simulink model "SlidesExampleNew_example"  (Simulink 7.4)
settings: Solver=FixedStepDiscrete  StartTime=0.0  StopTime=120  FixedStep=0.5  MaxStep=1  RelTol=1e-3
values from neighbouring files (symbols this model uses):
  y0 = -20    [SlidesExampleMfile.m]    (also in TrajectoryExampleScript.m)
libraries: BLOM_Lib x5
settings Model: Creator=vichik  LastModifiedBy=Kyle
settings OptimizationCC: BlockReduction=off  InitFltsAndDblsToZero=on
settings DebuggingCC: StrictBusMsg=ErrorLevel1

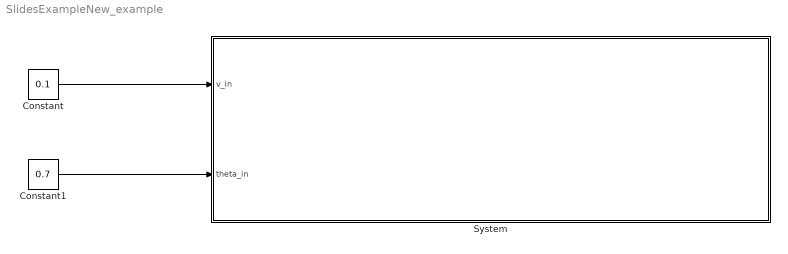
== system SlidesExampleNew_example ==
  Constant : Constant  Value=0.1
  Constant1 : Constant  Value=0.7
  System : Subsystem
  wires:
  Constant/1 -> System/1(v_in)
  Constant1/1 -> System/2(theta_in)

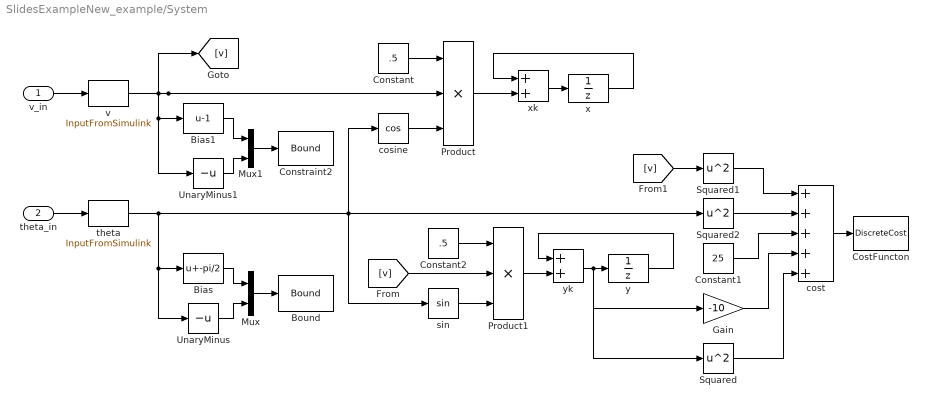
== system SlidesExampleNew_example/System ==
  v_in : Inport
  theta_in : Inport  Port=2
  Bias : Bias  Bias=-pi/2
  Bias1 : Bias  Bias=-1
  Bound : BLOM_Lib/Bound  SystemSampleTime=-1  ub=0  lb=-inf  initial_step=on  intermediate_step=on  final_step=on
  Constant : Constant  Value=.5  OutDataType=fixdt(1, 16)  OutScaling=2^0
  Constant1 : Constant  Value=25  OutDataType=fixdt(1, 16)  OutScaling=2^0
  Constant2 : Constant  Value=.5  OutDataType=fixdt(1, 16)  OutScaling=2^0
  Constraint2 : BLOM_Lib/Bound  SystemSampleTime=-1  ub=0  lb=-inf  initial_step=on  intermediate_step=on  final_step=on
  CostFuncton : BLOM_Lib/DiscreteCost  SystemSampleTime=-1  initial_step=on  intermediate_step=on  final_step=on
  Gain : Gain  Gain=-10  ParameterDataType=fixdt(1, 16)  ParameterScaling=2^0  OutDataType=fixdt(1, 16)  OutScaling=2^0
  Mux : Mux  Inputs=2
  Mux1 : Mux  Inputs=2
  Product : Product  Inputs=3  OutDataType=fixdt(1, 16)  OutScaling=2^0  RndMeth=Zero
  Product1 : Product  Inputs=***  OutDataType=fixdt(1, 16)  OutScaling=2^-10
  Squared : Math  Operator=square  OutDataType=fixdt(1, 16)  OutScaling=2^0  SaturateOnIntegerOverflow=on
  Squared1 : Math  Operator=square  OutDataType=fixdt(1, 16)  OutScaling=2^0  SaturateOnIntegerOverflow=on
  Squared2 : Math  Operator=square  OutDataType=fixdt(1, 16)  OutScaling=2^0  SaturateOnIntegerOverflow=on
  UnaryMinus : UnaryMinus
  UnaryMinus1 : UnaryMinus
  cosine : Trigonometry  Operator=cos
  cost : Sum  Inputs=5  OutDataType=fixdt(1, 16)  OutScaling=2^-10
  sin : Trigonometry
  theta : BLOM_Lib/InputFromSimulink  SystemSampleTime=-1  interpType=Zero-Order Hold
  v : BLOM_Lib/InputFromSimulink  SystemSampleTime=-1  interpType=Zero-Order Hold
  x : UnitDelay  SampleTime=-1
  xk : Sum  OutDataType=fixdt(1, 16)  OutScaling=2^-10
  y : UnitDelay  X0=y0  SampleTime=-1
  yk : Sum  OutDataType=fixdt(1, 16)  OutScaling=2^-10
  wires:
  x/1 -> xk/1
  v/1 -> UnaryMinus1/1, Bias1/1, [v], Product/2
  v_in/1 -> v/1
  theta_in/1 -> theta/1
  theta/1 -> cosine/1, Squared2/1, sin/1, UnaryMinus/1, Bias/1
  yk/1 -> Squared/1, Gain/1, y/1
  y/1 -> yk/1
  Bias/1 -> Mux/1
  UnaryMinus/1 -> Mux/2
  Bias1/1 -> Mux1/1
  UnaryMinus1/1 -> Mux1/2
  Mux1/1 -> Constraint2/1
  xk/1 -> x/1
  Product/1 -> xk/2
  cosine/1 -> Product/3
  Constant/1 -> Product/1
  Product1/1 -> yk/2
  sin/1 -> Product1/3
  Constant2/1 -> Product1/1
  cost/1 -> CostFuncton/1
  Squared1/1 -> cost/1
  Squared2/1 -> cost/2
  Constant1/1 -> cost/3
  Gain/1 -> cost/4
  Squared/1 -> cost/5
  [v] -> Product1/2
  [v] -> Squared1/1
  Mux/1 -> Bound/1
